simulink subsystem "Reference_curcle"  (R2024a)
settings: Solver=VariableStepAuto  StartTime=0.0  StopTime=10.0  RelTol=1e-3
undefined symbols (not defined in the file): circile_ref_amplitude, circile_ref_frequency
settings Model: Creator=tshintai  LastModifiedBy=tshintai
settings OptimizationCC: ReuseModelBlockBuffer=off
settings ModelReferenceCC: EnableRefExpFcnMdlSchedulingChecks=on
settings RTWCC: GPUComputeCapability=3.5

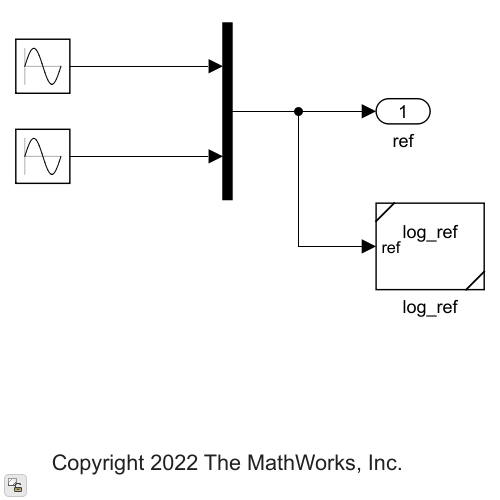
[thumbnail: Simulink's stored preview of the top-level diagram]
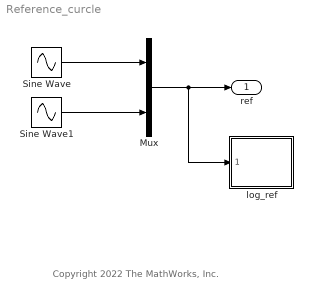
== system Reference_curcle ==
  note: Copyright 2022 The MathWorks, Inc.
  Mux : Mux  Inputs=2
  Sine Wave : Sin  Amplitude=circile_ref_amplitude  Frequency=circile_ref_frequency*2*pi  SampleTime=0
  Sine Wave1 : Sin  Amplitude=circile_ref_amplitude  Frequency=circile_ref_frequency*2*pi  Phase=pi/2  SampleTime=0
  log_ref : Subsystem  ReferencedSubsystem=log_ref
  ref : Outport
  wires:
  Sine Wave1/1 -> Mux/2
  Sine Wave/1 -> Mux/1
  Mux/1 -> log_ref/1, ref/1
